simulink model "MLC_LQR_Sim"  (R2019b)
settings: Solver=VariableStepAuto  StartTime=0.0  StopTime=20.0  RelTol=1e-3
values from neighbouring files (symbols this model uses):
  LQR_sys = ss(A,B,C,D)    [MLC_LQR_2.m]
undefined symbols (not defined in the file or in its folder): m_coeff
settings Model: Creator=idelafuentef  LastModifiedBy=idelafuentef

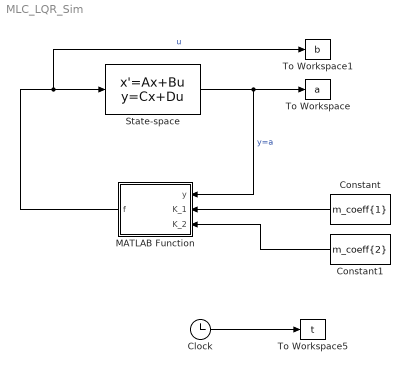
== system MLC_LQR_Sim ==
  Clock : Clock
      settings: Decimation=20
  Constant : Constant  Value=m_coeff{1}  VectorParams1D=off
  Constant1 : Constant  Value=m_coeff{2}  VectorParams1D=off
  MATLAB Function : MATLAB Function  TreatAsAtomicUnit=on
  State-space : StateSpace  A=LQR_sys.A  B=LQR_sys.B  C=LQR_sys.C  D=LQR_sys.D  InitialCondition=[1 0]
  To Workspace : ToWorkspace  VariableName=a  SaveFormat=Timeseries  SampleTime=-1
  To Workspace1 : ToWorkspace  VariableName=b  SaveFormat=Timeseries  SampleTime=-1
  To Workspace5 : ToWorkspace  VariableName=t  SaveFormat=Timeseries  SampleTime=-1
  wires:
  Clock/1 -> To Workspace5/1
  MATLAB Function/1(f) -> To Workspace1/1, State-space/1  "u"
  State-space/1 -> MATLAB Function/1(y), To Workspace/1  "y=a"
  Constant/1 -> MATLAB Function/2(K_1)
  Constant1/1 -> MATLAB Function/3(K_2)

== matlab function MLC_LQR_Sim/MATLAB Function ==
  data: y input; f output; K_1 input; K_2 input
function f = fcn(y,K_1,K_2)
    f=0;
    for i=1:length(K_1)
        f=f+K_1(i)*y(1)^(i-1);
    end
    for i=1:length(K_2)
        f=f+K_2(i)*y(2)^(i-1);
    end
end
